simulink model "TV_lisb"  (R2024b)
settings: Solver=ode45  StartTime=0.0  StopTime=10  MaxStep=0.05  RelTol=1e-3
model workspace: external: MATLAB File C:\Users\USER\Documents\MATLAB\NR\TV_lisb_helper_file.m (data not in the file)
values from neighbouring files (symbols this model uses):
  b = 0.1    [TV_lisb_helper_file.m]
  C1 = 1.28    [TV_lisb_helper_file.m]
  C2 = 23.99    [TV_lisb_helper_file.m]
  C3 = 0.52    [TV_lisb_helper_file.m]
  C_d = 0.89    [TV_lisb_helper_file.m]
  C_roll = 0.01    [TV_lisb_helper_file.m]
  frontal_area = 1.35    [TV_lisb_helper_file.m]
  g = 9.8    [TV_lisb_helper_file.m]
  I_w = 1.5    [TV_lisb_helper_file.m]
  Izz = 3000    [TV_lisb_helper_file.m]
  lf = 1.5    [TV_lisb_helper_file.m]
  lr = 1.5    [TV_lisb_helper_file.m]
  M = 300    [TV_lisb_helper_file.m]
  rho = 1.223    [TV_lisb_helper_file.m]
  tr = 1    [TV_lisb_helper_file.m]
  wr = 0.22    [TV_lisb_helper_file.m]
libraries: simulink x1
(part 2 of 2)

== system TV_lisb/Subsystem/Vertical Loads/F-z calcs/Term_2 ==
  hCG : Inport
  g : Inport  Port=2
  tr : Inport  Port=3
  tf : Inport  Port=4
  Acceleration_y : Inport  Port=5
  Add : Sum
  Add1 : Sum  Inputs=+-
  Add2 : Sum
  Add3 : Sum  Inputs=+-
  Constant : Constant  Value=0.5
  Divide : Product  Inputs=*/
  Divide1 : Product  Inputs=*/
  Divide2 : Product  Inputs=*/
  Product : Product
  Product1 : Product
  plus_f : Outport
  minus_f : Outport  Port=2
  plus_r : Outport  Port=3
  minus_r : Outport  Port=4
  wires:
  Add1/1 -> minus_f/1
  Add/1 -> plus_f/1
  hCG/1 -> Divide/1
  Add2/1 -> plus_r/1
  Add3/1 -> minus_r/1
  g/1 -> Divide/2
  Divide/1 -> Divide2/1, Divide1/1
  tf/1 -> Divide1/2
  Divide1/1 -> Product/1
  Acceleration_y/1 -> Product1/2, Product/2
  Product/1 -> Add/2, Add1/2
  Constant/1 -> Add3/1, Add1/1, Add2/1, Add/1
  tr/1 -> Divide2/2
  Divide2/1 -> Product1/1
  Product1/1 -> Add3/2, Add2/2

== system TV_lisb/Subsystem/Side Slip Angle/alpha1/tan_parameter/If Action Subsystem ==
  In1 : Inport
  Action Port : ActionPort  InitializeStates=reset  PropagateVarSize=During execution  ActionPortLabel=if(u1 == 0)
  Out1 : Outport
  wires:
  In1/1 -> Out1/1

== system TV_lisb/Subsystem/Side Slip Angle/alpha1/tan_parameter/If Action Subsystem1 ==
  Action Port : ActionPort  ActionPortLabel=else
  Constant : Constant  Value=0
  Out1 : Outport
  wires:
  Constant/1 -> Out1/1

== system TV_lisb/Subsystem/Side Slip Angle/alpha1/tan_parameter1/If Action Subsystem ==
  In1 : Inport
  Action Port : ActionPort  ActionPortLabel=if(u1 == 0)
  Out1 : Outport
  wires:
  In1/1 -> Out1/1

== system TV_lisb/Subsystem/Side Slip Angle/alpha1/tan_parameter1/If Action Subsystem1 ==
  Action Port : ActionPort  ActionPortLabel=else
  Constant : Constant  Value=0
  Out1 : Outport
  wires:
  Constant/1 -> Out1/1

== system TV_lisb/Subsystem/Side Slip Angle/alpha1/tan_parameter2/If Action Subsystem ==
  In1 : Inport
  Action Port : ActionPort  ActionPortLabel=if(u1 == 0)
  Out1 : Outport
  wires:
  In1/1 -> Out1/1

== system TV_lisb/Subsystem/Side Slip Angle/alpha1/tan_parameter2/If Action Subsystem1 ==
  Action Port : ActionPort  ActionPortLabel=else
  Constant : Constant  Value=0
  Out1 : Outport
  wires:
  Constant/1 -> Out1/1

== system TV_lisb/Subsystem/Side Slip Angle/alpha1/tan_parameter3/If Action Subsystem ==
  In1 : Inport
  Action Port : ActionPort  ActionPortLabel=if(u1 == 0)
  Out1 : Outport
  wires:
  In1/1 -> Out1/1

== system TV_lisb/Subsystem/Side Slip Angle/alpha1/tan_parameter3/If Action Subsystem1 ==
  Action Port : ActionPort  ActionPortLabel=else
  Constant : Constant  Value=0
  Out1 : Outport
  wires:
  Constant/1 -> Out1/1

== system TV_lisb/Subsystem/Slip Ratios/NaN handling/Subsystem/If Action Subsystem ==
  In1 : Inport
  Action Port : ActionPort  InitializeStates=reset  PropagateVarSize=During execution  ActionPortLabel=if(u1 == 0)
  Out1 : Outport
  wires:
  In1/1 -> Out1/1

== system TV_lisb/Subsystem/Slip Ratios/NaN handling/Subsystem/If Action Subsystem1 ==
  Action Port : ActionPort  ActionPortLabel=else
  Constant : Constant  Value=0
  Out1 : Outport
  wires:
  Constant/1 -> Out1/1

== system TV_lisb/Subsystem/Slip Ratios/NaN handling/Subsystem1/If Action Subsystem ==
  In1 : Inport
  Action Port : ActionPort  InitializeStates=reset  PropagateVarSize=During execution  ActionPortLabel=if(u1 == 0)
  Out1 : Outport
  wires:
  In1/1 -> Out1/1

== system TV_lisb/Subsystem/Slip Ratios/NaN handling/Subsystem1/If Action Subsystem1 ==
  Action Port : ActionPort  ActionPortLabel=else
  Constant : Constant  Value=0
  Out1 : Outport
  wires:
  Constant/1 -> Out1/1

== system TV_lisb/Subsystem/Slip Ratios/NaN handling/Subsystem2/If Action Subsystem ==
  In1 : Inport
  Action Port : ActionPort  InitializeStates=reset  PropagateVarSize=During execution  ActionPortLabel=if(u1 == 0)
  Out1 : Outport
  wires:
  In1/1 -> Out1/1

== system TV_lisb/Subsystem/Slip Ratios/NaN handling/Subsystem2/If Action Subsystem1 ==
  Action Port : ActionPort  ActionPortLabel=else
  Constant : Constant  Value=0
  Out1 : Outport
  wires:
  Constant/1 -> Out1/1

== system TV_lisb/Subsystem/Slip Ratios/NaN handling/Subsystem3/If Action Subsystem ==
  In1 : Inport
  Action Port : ActionPort  InitializeStates=reset  PropagateVarSize=During execution  ActionPortLabel=if(u1 == 0)
  Out1 : Outport
  wires:
  In1/1 -> Out1/1

== system TV_lisb/Subsystem/Slip Ratios/NaN handling/Subsystem3/If Action Subsystem1 ==
  Action Port : ActionPort  ActionPortLabel=else
  Constant : Constant  Value=0
  Out1 : Outport
  wires:
  Constant/1 -> Out1/1

== system TV_lisb/Subsystem/Tire Model/NaN handling/Subsystem/If Action Subsystem ==
  In1 : Inport
  Action Port : ActionPort  InitializeStates=reset  PropagateVarSize=During execution  ActionPortLabel=if(u1 == 0)
  Out1 : Outport
  wires:
  In1/1 -> Out1/1

== system TV_lisb/Subsystem/Tire Model/NaN handling/Subsystem/If Action Subsystem1 ==
  Action Port : ActionPort  ActionPortLabel=else
  Constant : Constant  Value=0
  Out1 : Outport
  wires:
  Constant/1 -> Out1/1

== system TV_lisb/Subsystem/Tire Model/NaN handling/Subsystem1/If Action Subsystem ==
  In1 : Inport
  Action Port : ActionPort  InitializeStates=reset  PropagateVarSize=During execution  ActionPortLabel=if(u1 == 0)
  Out1 : Outport
  wires:
  In1/1 -> Out1/1

== system TV_lisb/Subsystem/Tire Model/NaN handling/Subsystem1/If Action Subsystem1 ==
  Action Port : ActionPort  ActionPortLabel=else
  Constant : Constant  Value=0
  Out1 : Outport
  wires:
  Constant/1 -> Out1/1

== system TV_lisb/Subsystem/Tire Model/NaN handling/Subsystem2/If Action Subsystem ==
  In1 : Inport
  Action Port : ActionPort  InitializeStates=reset  PropagateVarSize=During execution  ActionPortLabel=if(u1 == 0)
  Out1 : Outport
  wires:
  In1/1 -> Out1/1

== system TV_lisb/Subsystem/Tire Model/NaN handling/Subsystem2/If Action Subsystem1 ==
  Action Port : ActionPort  ActionPortLabel=else
  Constant : Constant  Value=0
  Out1 : Outport
  wires:
  Constant/1 -> Out1/1

== system TV_lisb/Subsystem/Tire Model/NaN handling/Subsystem3/If Action Subsystem ==
  In1 : Inport
  Action Port : ActionPort  InitializeStates=reset  PropagateVarSize=During execution  ActionPortLabel=if(u1 == 0)
  Out1 : Outport
  wires:
  In1/1 -> Out1/1

== system TV_lisb/Subsystem/Tire Model/NaN handling/Subsystem3/If Action Subsystem1 ==
  Action Port : ActionPort  ActionPortLabel=else
  Constant : Constant  Value=0
  Out1 : Outport
  wires:
  Constant/1 -> Out1/1

== system TV_lisb/Subsystem/Tire Model/NaN handling1/Subsystem/If Action Subsystem ==
  In1 : Inport
  Action Port : ActionPort  InitializeStates=reset  PropagateVarSize=During execution  ActionPortLabel=if(u1 == 0)
  Out1 : Outport
  wires:
  In1/1 -> Out1/1

== system TV_lisb/Subsystem/Tire Model/NaN handling1/Subsystem/If Action Subsystem1 ==
  Action Port : ActionPort  ActionPortLabel=else
  Constant : Constant  Value=0
  Out1 : Outport
  wires:
  Constant/1 -> Out1/1

== system TV_lisb/Subsystem/Tire Model/NaN handling1/Subsystem1/If Action Subsystem ==
  In1 : Inport
  Action Port : ActionPort  InitializeStates=reset  PropagateVarSize=During execution  ActionPortLabel=if(u1 == 0)
  Out1 : Outport
  wires:
  In1/1 -> Out1/1

== system TV_lisb/Subsystem/Tire Model/NaN handling1/Subsystem1/If Action Subsystem1 ==
  Action Port : ActionPort  ActionPortLabel=else
  Constant : Constant  Value=0
  Out1 : Outport
  wires:
  Constant/1 -> Out1/1

== system TV_lisb/Subsystem/Tire Model/NaN handling1/Subsystem2/If Action Subsystem ==
  In1 : Inport
  Action Port : ActionPort  InitializeStates=reset  PropagateVarSize=During execution  ActionPortLabel=if(u1 == 0)
  Out1 : Outport
  wires:
  In1/1 -> Out1/1

== system TV_lisb/Subsystem/Tire Model/NaN handling1/Subsystem2/If Action Subsystem1 ==
  Action Port : ActionPort  ActionPortLabel=else
  Constant : Constant  Value=0
  Out1 : Outport
  wires:
  Constant/1 -> Out1/1

== system TV_lisb/Subsystem/Tire Model/NaN handling1/Subsystem3/If Action Subsystem ==
  In1 : Inport
  Action Port : ActionPort  InitializeStates=reset  PropagateVarSize=During execution  ActionPortLabel=if(u1 == 0)
  Out1 : Outport
  wires:
  In1/1 -> Out1/1

== system TV_lisb/Subsystem/Tire Model/NaN handling1/Subsystem3/If Action Subsystem1 ==
  Action Port : ActionPort  ActionPortLabel=else
  Constant : Constant  Value=0
  Out1 : Outport
  wires:
  Constant/1 -> Out1/1
